simulink model "METI_Thermal_ver01_Jmaab_2018b_Intg_Mref"  (R2018b)
settings: Solver=ode8  StartTime=0  StopTime=end_time  FixedStep=sampling_time  RelTol=1e-3
PreLoadFcn:
  | %init_setting;
values from neighbouring files (symbols this model uses):
  degC2K = 273.15    [METI_TRAMI_Thermal_ver01_Jmaab_PreLoad.m]    (also in init_setting_METI.m)
  K2degC = -273.15    [METI_TRAMI_Thermal_ver01_Jmaab_PreLoad.m]    (also in init_setting_METI.m)
  sampling_time = 0.0025    [METI_TRAMI_Thermal_ver01_Jmaab_PreLoad.m]
undefined symbols (not defined in the file or in its folder): ACC_D_Gain, ACC_I_Gain, ACC_P_Gain, ALT_CNT_ALT_OFF_RPM_HYS_rpm, ALT_CNT_ALT_ON_RPM_HYS_rpm, ALT_CNT_Alter_V_BASE_V, ALT_CNT_Alter_V_Kaisei_V, ALT_CNT_flag_disable_kaisei, ALT_CNT_V_Battely_Kudo_V, ALT_PNT_ALT_GDCurrent_A, ALT_PNT_ALT_GDVolt_V, ALT_PNT_Alter_limit_Current_V_table, ALT_PNT_Alter_limit_Current_V_table_x_rpm, ALT_PNT_Alter_trq_Nm_map, ALT_PNT_Alter_trq_Nm_map_x_rpm, ALT_PNT_Alter_trq_Nm_map_y_Current_A, ALT_PNT_Alter_trq_Nm_map_z_Volt_tgt_V, ALT_PNT_eta_pulley_alt, ALT_PNT_Gain_Alt_v_del, ALT_PNT_ratio_pulley_alt, ALT_PNT_Tau_Alternator_V_tgt_s, ALT_PNT_trq_alter_output_LL_Nm, BK_PNT_Pow_UL, BK_PNT_Tau_brake, Brk_LL, Brk_PGain, Brk_UL, BT_PNT_Lo_Capa_lo_batt_F, BT_PNT_Lo_ocv_SOC_lo_batt_OCV_V_table, BT_PNT_Lo_ocv_SOC_lo_batt_OCV_V_table_x_SOC, BT_PNT_Lo_R_lo_batt_ohm, BT_PNT_Lo_SOC_MAX_lo_batt, BT_PNT_Lo_SOC_MIN_lo_batt, BT_PNT_Lo_SOC_START_lo_batt, BT_PNT_Lo_V_start_ocv, DF_PNT_DF_gear, DF_PNT_Outtemp_degC, Driver_Brake_Const1, Driver_Brake_Const3, Driver_Brake_Switch_Const2, Driver_Brk_sh, drivmode_ACC, drivmode_CONST, drivmode_GensokuKaisei, drivmode_GensokuRikko, drivmode_STOP, EL_PNT_R_bodyelec_lo_ohm, ENG_CNT_acc_idlestop, ENG_CNT_Accel_LL, ENG_CNT_Accel_UL, ENG_CNT_brak_idlestop, ENG_CNT_flag_idle_stop_exe, ENG_CNT_gain_p_per_isc, ENG_CNT_IdleSpeed, ENG_CNT_IdleSpeed_Const, ENG_CNT_IdleStop_flag_const, ENG_CNT_omg_eng_fuelcut_rpm, ENG_CNT_per_isc_max, ENG_CNT_per_isc_min, ENG_CNT_per_throttle_fuelcut ... (+82)
libraries: METI_Lib_vehicle_model x18, simulink x3, AZAPA_Lib_vehicle_model x1
(part 1 of 3)
settings Model: Creator=nishimura  LastModifiedBy=E00026
settings DataIOCC: LimitDataPoints=on  SaveFormat=Array  InspectSignalLogs=on
settings OptimizationCC: BlockReduction=off  BooleanDataType=off  LifeSpan=inf
settings DebuggingCC: SaveWithParameterizedLinksMsg=none  UnderspecifiedInitializationDetection=Classic  MergeDetectMultiDrivingBlocksExec=none  SignalResolutionControl=TryResolveAllWithWarning  StrictBusMsg=ErrorOnBusTreatedAsVector  SFUnexpectedBacktrackingDiag=warning  SFNoUnconditionalDefaultTransitionDiag=warning  SFExecutionAtInitializationDiag=none
settings HardwareCC: ProdBitPerPointer=32  ProdBitPerSizeT=32  ProdBitPerPtrDiffT=32  ProdLargestAtomicFloat=None  ProdIntDivRoundTo=Undefined  ProdEndianess=Unspecified  ProdWordSize=32  ProdHWDeviceType=32-bit Generic  TargetUnknown=on
settings ModelReferenceCC: PropagateSignalLabelsOutOfModel=off
settings SFSimCC: SimUseLocalCustomCode=off
settings RTWCC: RTWUseLocalCustomCode=off
settings CodeAppCC: StateflowObjectComments=on
settings GRTTargetCC: TargetLangStandard=C89/C90 (ANSI)  GeneratePreprocessorConditionals=Disable all
settings ConfigComp: CovMetricSettings=dw  CovHtmlReporting=on  CovSaveCumulativeToWorkspaceVar=on  CovSaveSingleToWorkspaceVar=on  CovExternalEMLEnable=off  CovSFcnEnable=off

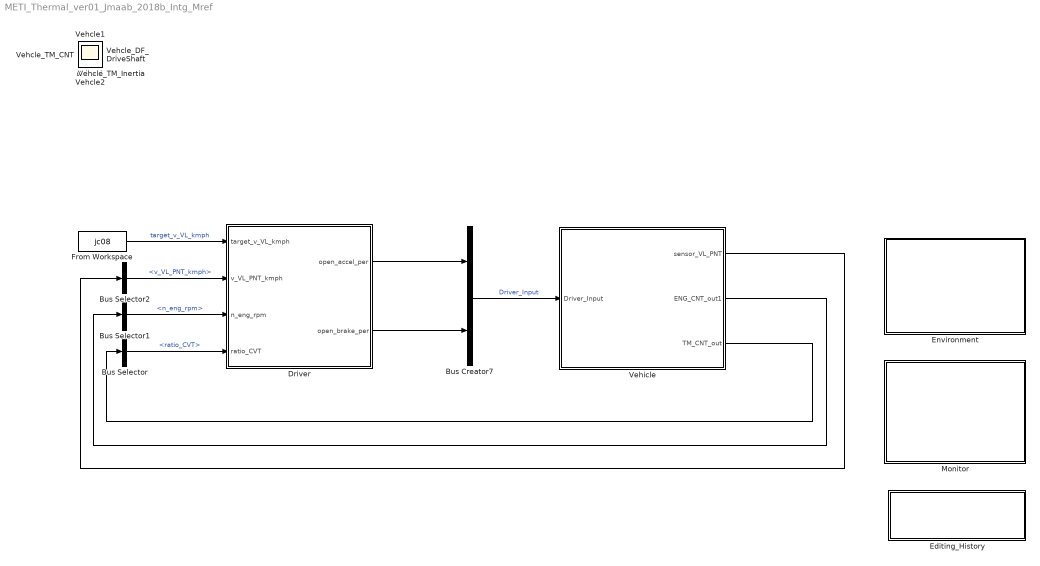
== system METI_Thermal_ver01_Jmaab_2018b_Intg_Mref ==
  Bus Creator7 : BusCreator  Inputs=2
  Bus Selector : BusSelector  OutputSignals=ratio_CVT
  Bus Selector1 : BusSelector  OutputSignals=n_eng_rpm
  Bus Selector2 : BusSelector  OutputSignals=v_VL_PNT_kmph
  Driver : Subsystem
      mask Display: image(imread('picture\ドライバ.png'))
  Editing_History : Subsystem
  Environment : Subsystem
      mask Display: image(imread('picture\外部環境.png'))
  From Workspace : FromWorkspace  VariableName=jc08  SampleTime=0  OutputAfterFinalValue=Holding final value
  Monitor : Subsystem
  Vehicle : Subsystem
      mask Display: image(imread('picture\電気負荷.png'))
  Driver1 : Scope
  Vehcle1 : Scope
  Vehcle2 : Scope
  Vehcle_DF_DriveShaft : Scope
  Vehcle_TM_CNT : Scope
  Vehcle_TM_Inertia : Scope
  wires:
  From Workspace/1 -> Driver/1(target_v_VL_kmph)  "target_v_VL_kmph"
  Bus Creator7/1 -> Vehicle/1(Driver_Input)  "Driver_Input"
  Vehicle/1(sensor_VL_PNT) -> Bus Selector2/1
  Vehicle/3(TM_CNT_out) -> Bus Selector/1
  Vehicle/2(ENG_CNT_out1) -> Bus Selector1/1
  Driver/1(open_accel_per) -> Bus Creator7/1
  Driver/2(open_brake_per) -> Bus Creator7/2
  Bus Selector/1 -> Driver/4(ratio_CVT)  "<ratio_CVT>"
  Bus Selector1/1 -> Driver/3(n_eng_rpm)  "<n_eng_rpm>"
  Bus Selector2/1 -> Driver/2(v_VL_PNT_kmph)  "<v_VL_PNT_kmph>"

== system METI_Thermal_ver01_Jmaab_2018b_Intg_Mref/Driver ==
  note: ドライバモデルのへたくそ対応
  note: 全体としてパワーを算出しておいて、
      | さらにパワーと速度のF/Bを切り替えれるようにしておく
  target_v_VL_kmph : Inport
  v_VL_PNT_kmph : Inport  Port=2
  n_eng_rpm : Inport  Port=3
  ratio_CVT : Inport  Port=4
  Caliculate_Driving_State : Subsystem
  Caliculate_Opeining_Accel : Subsystem
  Caliculate_Opening_Brake : Subsystem
  Memory2 : Memory  InheritSampleTime=on
  Memory3 : Memory
  Memory4 : Memory
  open_accel_per : Outport
  open_brake_per : Outport  Port=2
  tag scope: tScope_accel=global, tScope_brake=global
  wires:
  target_v_VL_kmph/1 -> Caliculate_Opening_Brake/2(target_v_VL_kmph), Caliculate_Driving_State/2(target_v_VL_kmph), Caliculate_Opeining_Accel/2(target_v_VL_kmph)
  Memory3/1 -> Caliculate_Opeining_Accel/3(pre_n_eng_rpm)  "pre_n_eng_rpm"
  ratio_CVT/1 -> Memory4/1
  Memory4/1 -> Caliculate_Opeining_Accel/4(pre_ratio_CVT)  "pre_ratio_CVT"
  n_eng_rpm/1 -> Memory3/1
  Memory2/1 -> Caliculate_Opening_Brake/1(v_VL_PNT_kmph), Caliculate_Opeining_Accel/1(v_VL_PNT_kmph)
  Caliculate_Opeining_Accel/1(open_accel_per) -> Caliculate_Opening_Brake/3(open_accel_per), open_accel_per/1, [tScope_accel]
  Caliculate_Opening_Brake/1(open_brake_per) -> Caliculate_Driving_State/1(open_brake_per), open_brake_per/1, [tScope_brake]
  v_VL_PNT_kmph/1 -> Memory2/1

== system METI_Thermal_ver01_Jmaab_2018b_Intg_Mref/Editing_History ==
  note: 編集履歴
      |
      | 2019/3/29　初版
      |
      | 2019/7/3　ver.2
      | ・ENG_CNT内部と出力の結線名を修正
      | ・DFとPTTH間の熱のI/Fを追加修正
      | ・PTTH_PNT/RDTH_PNTの絵が同梱されていなかったため追加

== system METI_Thermal_ver01_Jmaab_2018b_Intg_Mref/Environment ==
  note: 登坂。風、温度、湿度・・・
  Clock : Clock
  To Workspace : ToWorkspace  VariableName=simtime  SampleTime=-1
      settings: Decimation=num_tws_mabiki
  wires:
  Clock/1 -> To Workspace/1

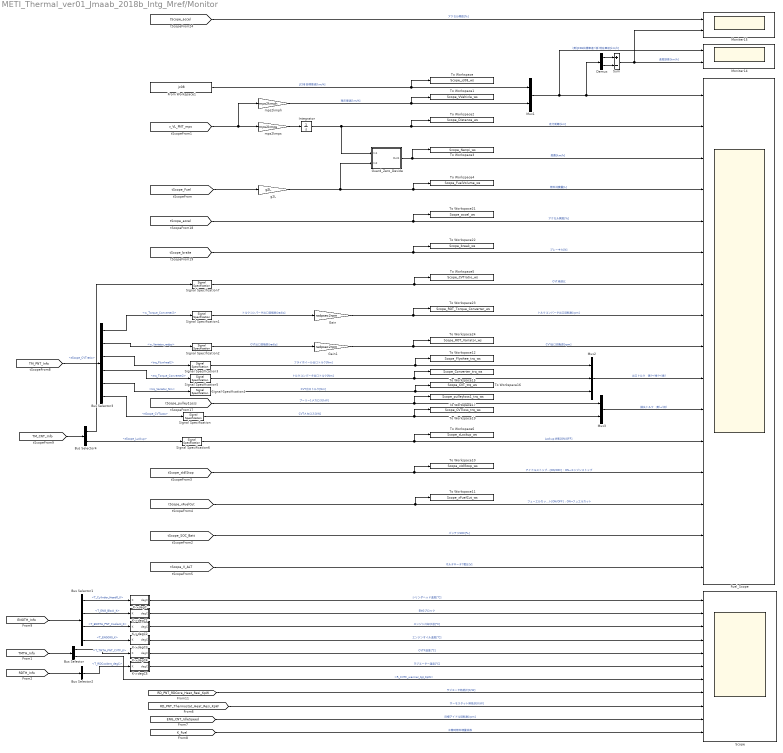
== system METI_Thermal_ver01_Jmaab_2018b_Intg_Mref/Monitor ==
  Bus Selector : BusSelector  OutputSignals=T_TMTH_PNT_CVTF_K,R_CVTF_warmer_tgt_KpW
  Bus Selector1 : BusSelector  OutputSignals=T_Cylinder_Head0_K,T_ENG_Block_K,T_ENGTH_PNT_Coolant_K,T_ENGOil0_K
  Bus Selector2 : BusSelector  OutputSignals=T_RDCoolant_degC
  Bus Selector3 : BusSelector  OutputSignals=w_Torque_Converter2,w_Variator_radps,trq_Flywheel2,trq_Torque_Converter2,trq_Variator_Nm,tScope_CVTLoss
  Bus Selector4 : BusSelector  OutputSignals=tScope_CVTratio,tScope_Luckup
  Demux : Demux  Outputs=2
  From Workspace1 : FromWorkspace  VariableName=jc08  SampleTime=0  OutputAfterFinalValue=Holding final value
  Fuel_Scope : Scope  NumInputPorts=16
  Gain : Gain  Gain=radpsec2rpm
  Gain1 : Gain  Gain=radpsec2rpm
  Guard_Zero_Devide : Subsystem
  Integrator : Integrator
  K->degC : Subsystem
  K->degC1 : Subsystem
  K->degC2 : Subsystem
  K->degC3 : Subsystem
  K->degC4 : Subsystem
  K->degC5 : Subsystem
  Moniter14 : Scope  NumInputPorts=2
  Moniter15 : Scope  NumInputPorts=2
  Mux1 : Mux  Inputs=2
  Mux2 : Mux  Inputs=3
  Mux3 : Mux  Inputs=2
  Scope : Scope  NumInputPorts=11
  Signal Specification{,1..7} (8 alike) : SignalSpecification
  Sum : Sum  Inputs=+-
  To Workspace : ToWorkspace  VariableName=Scope_jc08_ws  SaveFormat=Structure With Time  SampleTime=-1
      settings: Decimation=num_tws_mabiki
  To Workspace1 : ToWorkspace  VariableName=Scope_VVehicle_ws  SaveFormat=Structure With Time  SampleTime=-1
      settings: Decimation=num_tws_mabiki
  To Workspace10 : ToWorkspace  VariableName=Scope_xIdlStop_ws  SaveFormat=Structure With Time  SampleTime=-1
      settings: Decimation=num_tws_mabiki
  To Workspace11 : ToWorkspace  VariableName=Scope_xFuelCut_ws  SaveFormat=Structure With Time  SampleTime=-1
      settings: Decimation=num_tws_mabiki
  To Workspace12 : ToWorkspace  VariableName=Scope_Flywhee_trq_ws  SaveFormat=Structure With Time  SampleTime=-1
      settings: Decimation=num_tws_mabiki
  To Workspace15 : ToWorkspace  VariableName=Scope_Converter_trq_ws  SaveFormat=Structure With Time  SampleTime=-1
      settings: Decimation=num_tws_mabiki
  To Workspace16 : ToWorkspace  VariableName=Scope_CVT_trq_ws  SaveFormat=Structure With Time  SampleTime=-1
      settings: Decimation=num_tws_mabiki
  To Workspace17 : ToWorkspace  VariableName=Scope_pulleyloss1_trq_ws  SaveFormat=Structure With Time  SampleTime=-1
      settings: Decimation=num_tws_mabiki
  To Workspace19 : ToWorkspace  VariableName=Scope_CVTloss_trq_ws  SaveFormat=Structure With Time  SampleTime=-1
      settings: Decimation=num_tws_mabiki
  To Workspace2 : ToWorkspace  VariableName=Scope_Distance_ws  SaveFormat=Structure With Time  SampleTime=-1
      settings: Decimation=num_tws_mabiki
  To Workspace21 : ToWorkspace  VariableName=Scope_accel_ws  SaveFormat=Structure With Time  SampleTime=-1
      settings: Decimation=num_tws_mabiki
  To Workspace22 : ToWorkspace  VariableName=Scope_break_ws  SaveFormat=Structure With Time  SampleTime=-1
      settings: Decimation=num_tws_mabiki
  To Workspace23 : ToWorkspace  VariableName=Scope_ROT_Torque_Converter_ws  SaveFormat=Structure With Time  SampleTime=-1
      settings: Decimation=num_tws_mabiki
  To Workspace24 : ToWorkspace  VariableName=Scope_ROT_Variator_ws  SaveFormat=Structure With Time  SampleTime=-1
      settings: Decimation=num_tws_mabiki
  To Workspace3 : ToWorkspace  VariableName=Scope_Nenpi_ws  SaveFormat=Structure With Time  SampleTime=-1
      settings: Decimation=num_tws_mabiki
  To Workspace4 : ToWorkspace  VariableName=Scope_FuelVolume_ws  SaveFormat=Structure With Time  SampleTime=-1
      settings: Decimation=num_tws_mabiki
  To Workspace5 : ToWorkspace  VariableName=Scope_CVTratio_ws  SaveFormat=Structure With Time  SampleTime=-1
      settings: Decimation=num_tws_mabiki
  To Workspace6 : ToWorkspace  VariableName=Scope_xLockup_ws  SaveFormat=Structure With Time  SampleTime=-1
      settings: Decimation=num_tws_mabiki
  g2L : Gain  Gain=g2L
  mps2kmph : Gain  Gain=mps2kmph
  mps2kmps : Gain  Gain=mps2kmps
  wires:
  [tScope_xIdlStop] -> To Workspace10/1, Fuel_Scope/13  "アイドルストップ[ON/OFF] : ON→エンジンストップ"
  [tScope_xFuelCut] -> To Workspace11/1, Fuel_Scope/14  "フューエルカット[ON/OFF] : ON→フュエルカット"
  [v_VL_PNT_mps] -> mps2kmph/1, mps2kmps/1
  mps2kmps/1 -> Integrator/1
  [tScope_Fuel] -> g2L/1
  Integrator/1 -> Guard_Zero_Devide/1(In1), To Workspace2/1, Fuel_Scope/2  "走行距離[km]"
  g2L/1 -> To Workspace4/1, Fuel_Scope/4, Guard_Zero_Devide/2(In2)  "燃料消費量[L]"
  Signal Specification6/1 -> To Workspace6/1, Fuel_Scope/12  "Lockup状態[ON/OFF]"
  Signal Specification7/1 -> To Workspace5/1, Fuel_Scope/7  "CVT減速比"
  From Workspace1/1 -> To Workspace/1, Mux1/1  "JC08目標車速[km/h]"
  mps2kmph/1 -> To Workspace1/1, Mux1/2  "現在車速[km/h]"
  Mux1/1 -> Moniter14/1, Demux/1, Fuel_Scope/1  "(黄)JC08目標車速/(桃)現在車速[km/h]"
  Signal Specification/1 -> To Workspace19/1, Mux3/2  "CVTメカロス[kW]"
  Signal Specification3/1 -> To Workspace12/1, Mux2/1  "フライホイール出口トルク[Nm]"
  Signal Specification5/1 -> To Workspace15/1, Mux2/2  "トルクコンバータ出口トルク[Nm]"
  Signal Specification4/1 -> To Workspace16/1, Mux2/3  "CVT出口トルク[Nm]"
  [tScope_pulley1Loss] -> To Workspace17/1, Mux3/1  "プーリー1メカロス[kW]"
  Mux2/1 -> Fuel_Scope/10  "出口トルク  (黄)→(桃)→(青)"
  Mux3/1 -> Fuel_Scope/11  "損失トルク  (黄)→(桃)"
  [tScope_accel] -> To Workspace21/1, Fuel_Scope/5  "アクセル開度[%]"
  [tScope_brake] -> To Workspace22/1, Fuel_Scope/6  "ブレーキ力[N]"
  Gain/1 -> Fuel_Scope/8, To Workspace23/1  "トルクコンバータ出口回転数[rpm]"
  Signal Specification2/1 -> Gain1/1  "CVT出口回転数[rad/s]"
  Demux/1 -> Sum/1
  Demux/2 -> Sum/2
  Sum/1 -> Moniter14/2, Moniter15/2  "速度誤差[km/h]"
  [tScope_accel] -> Moniter15/1  "アクセル開度[%]"
  [tScope_V_ALT] -> Fuel_Scope/16  "オルタネータ7電圧[V]"
  [tScope_SOC_Batt] -> Fuel_Scope/15  "バッテリSOC[%]"
  Guard_Zero_Devide/1(Out1) -> To Workspace3/1, Fuel_Scope/3  "燃費[km/h]"
  K->degC4/1(degC) -> Scope/5  "CVTF温度[℃]"
  K->degC5/1(degC) -> Scope/6  "ラジエーター温度[℃]"
  K->degC2/1(degC) -> Scope/3  "エンジン冷却水温[℃]"
  K->degC3/1(degC) -> Scope/4  "エンジンオイル温度[℃]"
  K->degC/1(degC) -> Scope/1  "シリンダヘッド温度[℃]"
  K->degC1/1(degC) -> Scope/2  "ENGブロック"
  Signal Specification1/1 -> Gain/1  "トルクコンバータ出口回転数[rad/s]"
  Gain1/1 -> To Workspace24/1, Fuel_Scope/9  "CVT出口回転数[rpm]"
  [RD_PNT_RDCore_Heat_Resi_KpW] -> Scope/8  "ラジエータ熱抵抗[K/W]"
  [RD_PNT_Thermostat_Heat_Resi_KpW] -> Scope/9  "サーモスタット熱抵抗[K/W]"
  [ENG_CNT_IdleSpeed] -> Scope/10  "目標アイドル回転数[rpm]"
  [K_Fuel] -> Scope/11  "冷機時燃料増量係数"
  [ENGTH_Info] -> Bus Selector1/1
  Bus Selector1/1 -> K->degC/1(K)  "<T_Cylinder_Head0_K>"
  Bus Selector1/2 -> K->degC1/1(K)  "<T_ENG_Block_K>"
  Bus Selector1/3 -> K->degC2/1(K)  "<T_ENGTH_PNT_Coolant_K>"
  Bus Selector1/4 -> K->degC3/1(K)  "<T_ENGOil0_K>"
  [TMTH_Info] -> Bus Selector/1
  Bus Selector/1 -> K->degC4/1(K)  "<T_TMTH_PNT_CVTF_K>"
  [RDTH_Info] -> Bus Selector2/1
  Bus Selector2/1 -> K->degC5/1(K)  "<T_RDCoolant_degC>"
  Bus Selector/2 -> Scope/7  "<R_CVTF_warmer_tgt_KpW>"
  [TM_PNT_Info] -> Bus Selector3/1
  Bus Selector3/6 -> Signal Specification/1  "<tScope_CVTLoss>"
  Bus Selector3/1 -> Signal Specification1/1  "<w_Torque_Converter2>"
  Bus Selector3/2 -> Signal Specification2/1  "<w_Variator_radps>"
  Bus Selector3/3 -> Signal Specification3/1  "<trq_Flywheel2>"
  Bus Selector3/5 -> Signal Specification4/1  "<trq_Variator_Nm>"
  Bus Selector3/4 -> Signal Specification5/1  "<trq_Torque_Converter2>"
  [TM_CNT_Info] -> Bus Selector4/1
  Bus Selector4/2 -> Signal Specification6/1  "<tScope_Luckup>"
  Bus Selector4/1 -> Signal Specification7/1  "<tScope_CVTratio>"

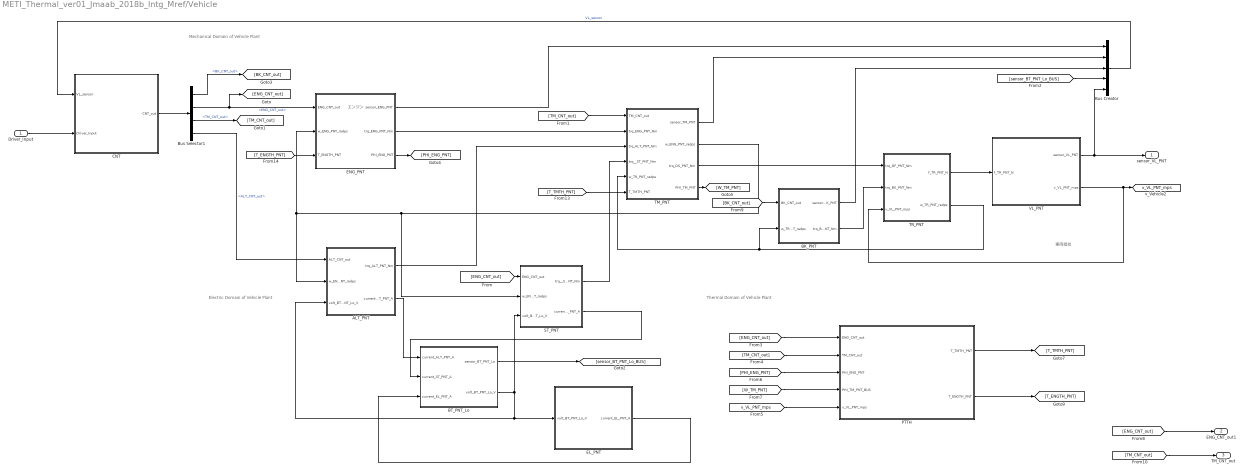
== system METI_Thermal_ver01_Jmaab_2018b_Intg_Mref/Vehicle ==
  note: Thermal Domain of Vehicle Plant
  note: エンジン
  note: 車両抵抗
  note: Mechanical Domain of Vehicle Plant
  note: Electric Domain
      |  of Vehicle Plant
  Driver_Input : Inport
  ALT_PNT : Subsystem
      mask Display: image(imread('picture\image\オルタネータ02.jpg'))
  BK_PNT : Subsystem
      mask Display: image(imread('picture\ブレーキ02.png'))
  BT_PNT_Lo : Subsystem
      mask Display: image(imread('picture\バッテリー.png'))
  Bus Creator : BusCreator  Inputs=5
  Bus Selector1 : BusSelector  OutputSignals=BK_CNT_out,ENG_CNT_out,TM_CNT_out,ALT_CNT_out
  CNT : Subsystem
      mask Display: image(imread('picture\ECU.png'))
  EL_PNT : Subsystem
      mask Display: image(imread('picture\電気負荷.png'))
  ENG_PNT : Subsystem
      mask Display: image(imread('picture\image\エンジン03.jpg'))
  PTTH : Subsystem
  ST_PNT : Subsystem
      mask Display: image(imread('picture\image\スターター02.jpg'))
  TM_PNT : Subsystem
      mask Display: image(imread('picture\image\トランスミッション02.jpg'))
  TR_PNT : Subsystem
      mask Display: image(imread('picture\タイヤ01.png'))
  VL_PNT : Subsystem
      mask Display: image(imread('picture\車両抵抗.png'))
  sensor_VL_PNT : Outport
  ENG_CNT_out1 : Outport  Port=2
  TM_CNT_out : Outport  Port=3
  tag scope: v_VL_PNT_mps=global
  wires:
  ALT_PNT/1(trq_ALT_PNT_Nm) -> TM_PNT/3(trq_ALT_PNT_Nm)
  EL_PNT/1(current_EL_PNT_A) -> BT_PNT_Lo/3(current_EL_PNT_A)
  ALT_PNT/2(current_ALT_PNT_A) -> BT_PNT_Lo/1(current_ALT_PNT_A)
  ST_PNT/2(current_ST_PNT_A) -> BT_PNT_Lo/2(current_ST_PNT_A)
  BT_PNT_Lo/2(volt_BT_PNT_Lo_V) -> ST_PNT/3(volt_BT_PNT_Lo_V), ALT_PNT/3(volt_BT_PNT_Lo_V), EL_PNT/1(volt_BT_PNT_Lo_V)
  ENG_PNT/2(trq_ENG_PNT_Nm) -> TM_PNT/2(trq_ENG_PNT_Nm)
  ST_PNT/1(trq__ST_PNT_Nm) -> TM_PNT/4(trq__ST_PNT_Nm)
  VL_PNT/1(sensor_VL_PNT) -> Bus Creator/5, sensor_VL_PNT/1
  BK_PNT/2(trq_BK_PNT_Nm) -> TR_PNT/2(trq_BK_PNT_Nm)
  TR_PNT/1(f_TR_PNT_N) -> VL_PNT/1(f_TR_PNT_N)
  TR_PNT/2(w_TR_PNT_radps) -> BK_PNT/2(w_TR_PNT_radps), TM_PNT/5(w_TR_PNT_radps)
  VL_PNT/2(v_VL_PNT_mps) -> TR_PNT/3(v_VL_PNT_mps), [v_VL_PNT_mps]
  [TM_CNT_out] -> TM_CNT_out/1
  Bus Selector1/2 -> [ENG_CNT_out], ENG_PNT/1(ENG_CNT_out)  "<ENG_CNT_out>"
  Bus Selector1/4 -> ALT_PNT/1(ALT_CNT_out)  "<ALT_CNT_out>"
  CNT/1(CNT_out) -> Bus Selector1/1
  [ENG_CNT_out] -> ST_PNT/1(ENG_CNT_out)
  Bus Selector1/3 -> [TM_CNT_out]  "<TM_CNT_out>"
  [TM_CNT_out] -> TM_PNT/1(TM_CNT_out)
  BT_PNT_Lo/1(sensor_BT_PNT_Lo) -> [sensor_BT_PNT_Lo_BUS]
  Driver_Input/1 -> CNT/2(Driver_Input)
  [ENG_CNT_out] -> ENG_CNT_out1/1
  TM_PNT/3(trq_DS_PNT_Nm) -> TR_PNT/1(trq_DF_PNT_Nm)
  [T_TMTH_PNT] -> TM_PNT/6(T_TMTH_PNT)
  [v_VL_PNT_mps] -> PTTH/5(v_VL_PNT_mps)
  [ENG_CNT_out] -> PTTH/1(ENG_CNT_out)
  [TM_CNT_out] -> PTTH/2(TM_CNT_out)
  ENG_PNT/3(PHI_ENG_PNT) -> [PHI_ENG_PNT]
  [PHI_ENG_PNT] -> PTTH/3(PHI_ENG_PNT)
  [W_TM_PNT] -> PTTH/4(PHI_TM_PNT_BUS)
  TM_PNT/4(PHI_TM_PNT) -> [W_TM_PNT]
  PTTH/1(T_TMTH_PNT) -> [T_TMTH_PNT]
  PTTH/2(T_ENGTH_PNT) -> [T_ENGTH_PNT]
  [T_ENGTH_PNT] -> ENG_PNT/3(T_ENGTH_PNT)
  [sensor_BT_PNT_Lo_BUS] -> Bus Creator/4
  ENG_PNT/1(sensor_ENG_PNT) -> Bus Creator/1
  TM_PNT/1(sensor_TM_PNT) -> Bus Creator/2
  Bus Selector1/1 -> [BK_CNT_out]  "<BK_CNT_out>"
  [BK_CNT_out] -> BK_PNT/1(BK_CNT_out)
  Bus Creator/1 -> CNT/1(VL_sensor)  "VL_sensor"
  TM_PNT/2(w_ENG_PNT_radps) -> ENG_PNT/2(w_ENG_PNT_radps), ALT_PNT/2(w_ENG_PNT_radps), ST_PNT/2(w_ENG_PNT_radps)
  BK_PNT/1(sensor_BK_PNT) -> Bus Creator/3

== system METI_Thermal_ver01_Jmaab_2018b_Intg_Mref/Driver/Caliculate_Driving_State ==
  open_brake_per : Inport
  target_v_VL_kmph : Inport  Port=2
  Constant : Constant  Value=Thresh_Stop_vCar
  Constant4 : Constant  Value=0.1*sampling_time
  Constant6 : Constant  Value=-0.1*sampling_time
  Memory : Memory
  Relational Operator : RelationalOperator  Operator=>  OutDataTypeStr=boolean  RndMeth=Nearest
  Relational Operator1 : RelationalOperator  Operator=<  OutDataTypeStr=boolean  RndMeth=Nearest
  Relational Operator2 : RelationalOperator  Operator=<  OutDataTypeStr=boolean  RndMeth=Nearest
  Sum : Sum  Inputs=|+-
  Switch{,1..3} (4 alike) : Switch  Criteria=u2 > Threshold  Threshold=0.5
  Terminator : Terminator
  停止 : Constant  Value=drivmode_STOP
  加速 : Constant  Value=drivmode_ACC
  定常1 : Constant  Value=drivmode_CONST
  減速力行 : Constant  Value=drivmode_GensokuRikko
  減速回生 : Constant  Value=drivmode_GensokuKaisei
  wires:
  Switch/1 -> Terminator/1  "state_driving"
  target_v_VL_kmph/1 -> Relational Operator/1, Memory/1, Sum/1
  Relational Operator1/1 -> Switch1/2
  Constant4/1 -> Relational Operator1/2
  Relational Operator/1 -> Switch/2
  Constant/1 -> Relational Operator/2
  停止/1 -> Switch/3
  Sum/1 -> Relational Operator1/1, Relational Operator2/1
  減速回生/1 -> Switch2/1
  Switch3/1 -> Switch1/1
  Constant6/1 -> Relational Operator2/2
  Memory/1 -> Sum/2
  open_brake_per/1 -> Switch2/2
  減速力行/1 -> Switch2/3
  Relational Operator2/1 -> Switch3/2
  Switch2/1 -> Switch3/1
  定常1/1 -> Switch3/3
  加速/1 -> Switch1/3
  Switch1/1 -> Switch/1

== system METI_Thermal_ver01_Jmaab_2018b_Intg_Mref/Driver/Caliculate_Opeining_Accel ==
  v_VL_PNT_kmph : Inport
  target_v_VL_kmph : Inport  Port=2
  pre_n_eng_rpm : Inport  Port=3
  pre_ratio_CVT : Inport  Port=4
  FB : Subsystem  mask{P_Gain=ACC_P_Gain, D_Gain=ACC_D_Gain, I_Gain=ACC_I_Gain}
      mask prompts: P_Gain "Pゲイン値"; D_Gain "Dゲイン値"; I_Gain "Iゲイン値"
  FF : Subsystem
  Guard_0_100 : Saturate  UpperLimit=ENG_CNT_Throttle_UL  LowerLimit=ENG_CNT_Throttle_LL
  Sum1 : Sum  Inputs=|-+
  Sum3 : Sum  Inputs=++|
  open_accel_per : Outport
  wires:
  Sum1/1 -> FB/1(delta_v_VL_kmph)
  v_VL_PNT_kmph/1 -> FF/1(v_VL_PNT_kmph), Sum1/1
  target_v_VL_kmph/1 -> FF/2(target_v_VL_kmph), Sum1/2
  Sum3/1 -> Guard_0_100/1
  pre_n_eng_rpm/1 -> FF/3(pre_n_eng_rpm)
  pre_ratio_CVT/1 -> FF/4(pre_ratio_CVT)
  FB/1(FB_open_accel_per) -> Sum3/1
  FF/1(FF_open_accel_per) -> Sum3/2
  Guard_0_100/1 -> open_accel_per/1  "open_accel_per"

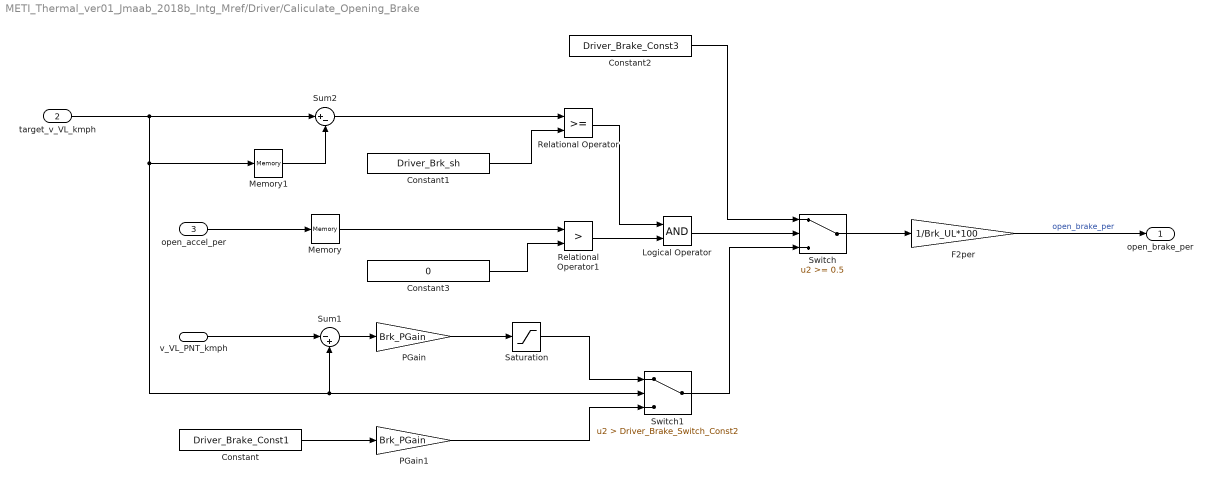
== system METI_Thermal_ver01_Jmaab_2018b_Intg_Mref/Driver/Caliculate_Opening_Brake ==
  v_VL_PNT_kmph : Inport
  target_v_VL_kmph : Inport  Port=2
  open_accel_per : Inport  Port=3
  Constant : Constant  Value=Driver_Brake_Const1
  Constant1 : Constant  Value=Driver_Brk_sh
  Constant2 : Constant  Value=Driver_Brake_Const3
  Constant3 : Constant  Value=0
  F2per : Gain  Gain=1/Brk_UL*100
  Logical Operator : Logic  AllPortsSameDT=off  OutDataTypeStr=boolean
  Memory : Memory
  Memory1 : Memory
  PGain : Gain  Gain=Brk_PGain
  PGain1 : Gain  Gain=Brk_PGain
  Relational Operator : RelationalOperator  OutDataTypeStr=boolean  RndMeth=Nearest
  Relational Operator1 : RelationalOperator  Operator=>  OutDataTypeStr=boolean  RndMeth=Nearest
  Saturation : Saturate  UpperLimit=Brk_UL  LowerLimit=Brk_LL
  Sum1 : Sum  Inputs=|-+
  Sum2 : Sum  Inputs=|+-
  Switch : Switch  Threshold=0.5
  Switch1 : Switch  Criteria=u2 > Threshold  Threshold=Driver_Brake_Switch_Const2
  open_brake_per : Outport
  wires:
  target_v_VL_kmph/1 -> Switch1/2, Sum1/2, Memory1/1, Sum2/1
  Sum1/1 -> PGain/1
  PGain/1 -> Saturation/1
  Constant/1 -> PGain1/1
  PGain1/1 -> Switch1/3
  open_accel_per/1 -> Memory/1
  Memory/1 -> Relational Operator1/1
  Memory1/1 -> Sum2/2
  Switch/1 -> F2per/1
  Sum2/1 -> Relational Operator/1
  Saturation/1 -> Switch1/1
  Switch1/1 -> Switch/3
  Constant2/1 -> Switch/1
  v_VL_PNT_kmph/1 -> Sum1/1
  Constant1/1 -> Relational Operator/2
  Constant3/1 -> Relational Operator1/2
  Relational Operator1/1 -> Logical Operator/2
  Relational Operator/1 -> Logical Operator/1
  Logical Operator/1 -> Switch/2
  F2per/1 -> open_brake_per/1  "open_brake_per"

== system METI_Thermal_ver01_Jmaab_2018b_Intg_Mref/Monitor/Guard_Zero_Devide ==
  note: 0割防止暫定処置
  In1 : Inport
  In2 : Inport  Port=2
  Constant1 : Constant  Value=fuel_0guard
  Constant2 : Constant  Value=fuelcomsnp_0
  Divide : Product  Inputs=*/
  MinMax : MinMax  Function=max  Inputs=2
  Relational Operator : RelationalOperator  OutDataTypeStr=boolean  RndMeth=Nearest
  Switch1 : Switch  Criteria=u2 > Threshold  Threshold=0.5
  Out1 : Outport
  wires:
  In2/1 -> MinMax/1, Relational Operator/1
  In1/1 -> Divide/1
  Switch1/1 -> Out1/1  "燃費[km/l]"
  Divide/1 -> Switch1/1  "燃費[km/l]"
  Constant2/1 -> Switch1/3
  Relational Operator/1 -> Switch1/2
  MinMax/1 -> Divide/2
  Constant1/1 -> MinMax/2, Relational Operator/2

== system METI_Thermal_ver01_Jmaab_2018b_Intg_Mref/Monitor/K->degC ==
  K : Inport
  Constant2 : Constant  Value=K2degC
  Sum : Sum  Inputs=++|
  degC : Outport
  wires:
  Sum/1 -> degC/1
  Constant2/1 -> Sum/1
  K/1 -> Sum/2

== system METI_Thermal_ver01_Jmaab_2018b_Intg_Mref/Monitor/K->degC1 ==
  K : Inport
  Constant2 : Constant  Value=K2degC
  Sum : Sum  Inputs=++|
  degC : Outport
  wires:
  K/1 -> Sum/2
  Constant2/1 -> Sum/1
  Sum/1 -> degC/1

== system METI_Thermal_ver01_Jmaab_2018b_Intg_Mref/Monitor/K->degC2 ==
  K : Inport
  Constant2 : Constant  Value=K2degC
  Sum : Sum  Inputs=++|
  degC : Outport
  wires:
  Sum/1 -> degC/1
  Constant2/1 -> Sum/1
  K/1 -> Sum/2

== system METI_Thermal_ver01_Jmaab_2018b_Intg_Mref/Monitor/K->degC3 ==
  K : Inport
  Constant2 : Constant  Value=K2degC
  Sum : Sum  Inputs=++|
  degC : Outport
  wires:
  K/1 -> Sum/2
  Constant2/1 -> Sum/1
  Sum/1 -> degC/1

== system METI_Thermal_ver01_Jmaab_2018b_Intg_Mref/Monitor/K->degC4 ==
  K : Inport
  Constant2 : Constant  Value=K2degC
  Sum : Sum  Inputs=++|
  degC : Outport
  wires:
  Sum/1 -> degC/1
  Constant2/1 -> Sum/1
  K/1 -> Sum/2

== system METI_Thermal_ver01_Jmaab_2018b_Intg_Mref/Monitor/K->degC5 ==
  K : Inport
  Constant2 : Constant  Value=K2degC
  Sum : Sum  Inputs=++|
  degC : Outport
  wires:
  K/1 -> Sum/2
  Constant2/1 -> Sum/1
  Sum/1 -> degC/1

== system METI_Thermal_ver01_Jmaab_2018b_Intg_Mref/Vehicle/ALT_PNT ==
  note: 発電する為のトルクが負
  note: スルー量が出力の場合、発電する方向が正
  ALT_CNT_out : Inport
  w_ENG_PNT_radps : Inport  Port=2
  volt_BT_PNT_Lo_V : Inport  Port=3
  Bus Selector8 : BusSelector  OutputSignals=target_volt_ALT_V
  Gain : Gain  Gain=-1
  Memory1 : Memory
  P_cal : METI_Lib_vehicle_model/P_cal  Type_energy=回転運動  Type_output_energy=出力  Power_name=Po_  t_Workspace_Name=ALT_PNT_MECK  P_VariableName=Po_ALT_PNT_MECK  Across_VariableName=w_ALT_PNT_MECK  Throgh_VariableName=tq_ALT_PNT_MECK
  P_cal1 : METI_Lib_vehicle_model/P_cal  Type_energy=電気  Type_output_energy=出力  Power_name=Po_  t_Workspace_Name=ALT_PNT_ELEC  P_VariableName=Po_ALT_PNT_ELEC  Across_VariableName=V_ALT_PNT_ELEC  Throgh_VariableName=I_ALT_PNT_ELEC
  Subsystem : Subsystem
  Terminator : Terminator
  Terminator1 : Terminator
  pulley_slave : Subsystem
  trq_ALT_PNT_Nm : Outport
  current_ALT_PNT_A : Outport  Port=2
  tag scope: tScope_V_ALT=global
  wires:
  Memory1/1 -> Subsystem/2(w_ROT_slavepulley12)
  Subsystem/1(current_ALT_PNT_A) -> P_cal1/2, current_ALT_PNT_A/1
  Gain/1 -> trq_ALT_PNT_Nm/1  "trq_ALT_PNT_Nm"
  pulley_slave/1(trq_slavepulley11) -> Gain/1
  w_ENG_PNT_radps/1 -> pulley_slave/1(w_ENG_PNT_radps)
  Subsystem/2(trq_trqsource) -> P_cal/2, pulley_slave/2(trq_slavepulley12)
  volt_BT_PNT_Lo_V/1 -> [tScope_V_ALT], P_cal1/1, Subsystem/3(volt_BT_PNT_Lo_V)
  P_cal1/1 -> Terminator1/1
  P_cal/1 -> Terminator/1
  pulley_slave/2(w_slavepulley12) -> P_cal/1, Memory1/1
  ALT_CNT_out/1 -> Bus Selector8/1
  Bus Selector8/1 -> Subsystem/1(target_volt_ALT_V)  "<target_volt_ALT_V>"

== system METI_Thermal_ver01_Jmaab_2018b_Intg_Mref/Vehicle/BK_PNT ==
  note: 制動力
  BK_CNT_out : Inport
  w_TR_PNT_radps : Inport  Port=2
  Bus Creator : BusCreator  Inputs=1
  Bus Selector : BusSelector  OutputSignals=open_brake_per
  Constant2 : Constant  Value=tire_r
  Gain : Gain  Gain=-1
  Memory : Memory
  Product6 : Product  RndMeth=Zero
  Q_cal3 : METI_Lib_vehicle_model/P_cal  Type_energy=回転運動  Type_output_energy=損失  Power_name=Pl_  t_Workspace_Name=BK_PNT_MECK_LOSS  P_VariableName=Pl_BK_PNT_MECK_LOSS  Across_VariableName=w_BK_PNT_MECK_LOSS  Throgh_VariableName=tq_BK_PNT_MECK_LOSS
  Terminator1 : Terminator
  Transfer Fcn : TransferFcn  Denominator=[BK_PNT_Tau_brake 1]
  per2F : Gain  Gain=BK_PNT_Pow_UL/100
  sensor_BK_PNT : Outport
  trq_BK_PNT_Nm : Outport  Port=2
  wires:
  Q_cal3/1 -> Terminator1/1
  Transfer Fcn/1 -> Product6/2
  Constant2/1 -> Product6/1
  Product6/1 -> Gain/1, Q_cal3/2
  w_TR_PNT_radps/1 -> Q_cal3/1
  BK_CNT_out/1 -> Bus Selector/1
  Gain/1 -> Bus Creator/1, trq_BK_PNT_Nm/1  "trq_BK_PNT_Nm"
  per2F/1 -> Transfer Fcn/1
  Bus Selector/1 -> per2F/1  "<open_brake_per>"
  Memory/1 -> sensor_BK_PNT/1  "sensor_BK_PNT"
  Bus Creator/1 -> Memory/1

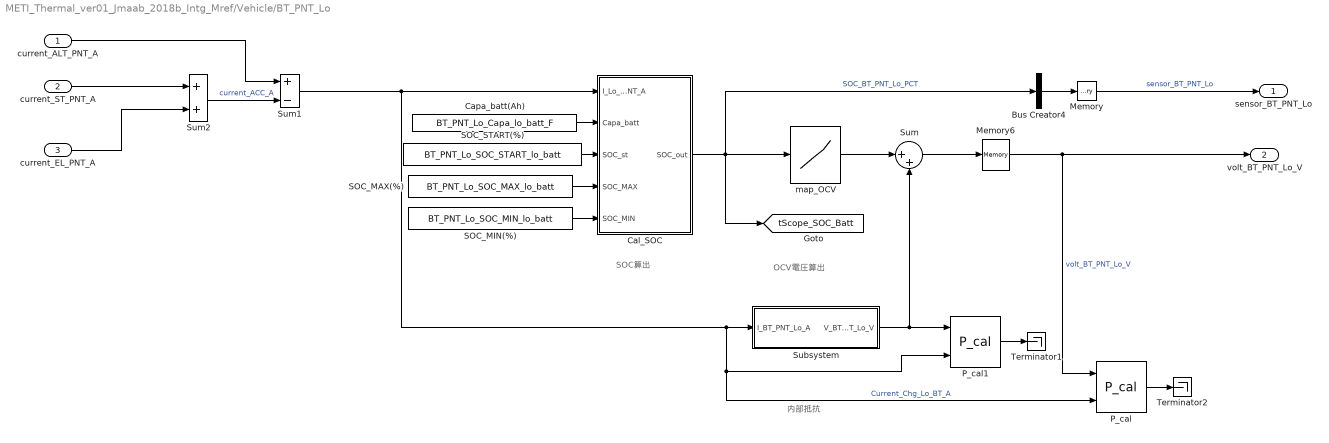
== system METI_Thermal_ver01_Jmaab_2018b_Intg_Mref/Vehicle/BT_PNT_Lo ==
  note: SOC算出
  note: 内部抵抗
  note: OCV電圧算出
  current_ALT_PNT_A : Inport
  current_ST_PNT_A : Inport  Port=2
  current_EL_PNT_A : Inport  Port=3
  Bus Creator4 : BusCreator  Inputs=1
  Cal_SOC : Subsystem
  Capa_batt(Ah) : Constant  Value=BT_PNT_Lo_Capa_lo_batt_F
  Memory : Memory
  Memory6 : Memory  InitialCondition=BT_PNT_Lo_V_start_ocv  InheritSampleTime=on
  P_cal : METI_Lib_vehicle_model/P_cal  Type_energy=電気  Type_output_energy=出力  Power_name=Po_  t_Workspace_Name=BT_PNT_Lo_ELEC  P_VariableName=Po_BT_PNT_Lo_ELEC  Across_VariableName=V_BT_PNT_Lo_ELEC  Throgh_VariableName=I_BT_PNT_Lo_ELEC
  P_cal1 : METI_Lib_vehicle_model/P_cal  Type_energy=電気  Type_output_energy=損失  Power_name=Pl_  t_Workspace_Name=BT_PNT_Lo_ELEC_LOSS  P_VariableName=Pl_BT_PNT_Lo_ELEC_LOSS  Across_VariableName=V_BT_PNT_Lo_ELEC_LOSS  Throgh_VariableName=I_BT_PNT_Lo_ELEC_LOSS
  SOC_MAX(%) : Constant  Value=BT_PNT_Lo_SOC_MAX_lo_batt
  SOC_MIN(%) : Constant  Value=BT_PNT_Lo_SOC_MIN_lo_batt
  SOC_START(%) : Constant  Value=BT_PNT_Lo_SOC_START_lo_batt
  Subsystem : Subsystem
  Sum : Sum  Inputs=|++
  Sum1 : Sum  Inputs=+-
  Sum2 : Sum
  Terminator1 : Terminator
  Terminator2 : Terminator
  map_OCV : Lookup  InputValues=BT_PNT_Lo_ocv_SOC_lo_batt_OCV_V_table_x_SOC  Table=BT_PNT_Lo_ocv_SOC_lo_batt_OCV_V_table  LookUpMeth=Interpolation-Use End Values
  sensor_BT_PNT_Lo : Outport
  volt_BT_PNT_Lo_V : Outport  Port=2
  tag scope: tScope_SOC_Batt=global
  wires:
  Sum/1 -> Memory6/1
  Capa_batt(Ah)/1 -> Cal_SOC/2(Capa_batt)
  SOC_START(%)/1 -> Cal_SOC/3(SOC_st)
  SOC_MAX(%)/1 -> Cal_SOC/4(SOC_MAX)
  SOC_MIN(%)/1 -> Cal_SOC/5(SOC_MIN)
  Memory6/1 -> volt_BT_PNT_Lo_V/1, P_cal/1  "volt_BT_PNT_Lo_V"
  map_OCV/1 -> Sum/1
  Subsystem/1(V_BT_PNT_Lo_V) -> P_cal1/1, Sum/2
  P_cal/1 -> Terminator2/1
  P_cal1/1 -> Terminator1/1
  Cal_SOC/1(SOC_out) -> Bus Creator4/1, map_OCV/1, [tScope_SOC_Batt]  "SOC_BT_PNT_Lo_PCT"
  Memory/1 -> sensor_BT_PNT_Lo/1  "sensor_BT_PNT_Lo"
  Sum1/1 -> P_cal/2, P_cal1/2, Subsystem/1(I_BT_PNT_Lo_A), Cal_SOC/1(I_Lo_BT_PNT_A)  "Current_Chg_Lo_BT_A"
  Sum2/1 -> Sum1/2  "current_ACC_A"
  current_ALT_PNT_A/1 -> Sum1/1
  current_ST_PNT_A/1 -> Sum2/1
  current_EL_PNT_A/1 -> Sum2/2
  Bus Creator4/1 -> Memory/1

== system METI_Thermal_ver01_Jmaab_2018b_Intg_Mref/Vehicle/CNT ==
  note: Control Model
  note: Gtoto From Tag Visibility for CAN
  VL_sensor : Inport
  Driver_Input : Inport  Port=2
  ALT_CNT : Subsystem
  BK_CNT : Subsystem
  Bus Creator1 : BusCreator  Inputs=4
  Bus Selector : BusSelector  OutputSignals=sensor_ENG_PNT,sensor_TM_PNT,sensor_BT_PNT_Lo,sensor_VL_PNT,sensor_BK_PNT
  CAN : Subsystem
  ENG_CNT : Subsystem
  Goto Tag Visibility : GotoTagVisibility  GotoTag=ENG_CNT_CAN_Tx
  Goto Tag Visibility1 : GotoTagVisibility  GotoTag=TM_CNT_CAN_Tx
  Goto Tag Visibility2 : GotoTagVisibility  GotoTag=ALT_CNT_CAN_Rx
  Goto Tag Visibility3 : GotoTagVisibility  GotoTag=ENG_CNT_CAN_Rx
  Goto Tag Visibility4 : GotoTagVisibility  GotoTag=TM_CNT_CAN_Rx
  Goto Tag Visibility5 : GotoTagVisibility  GotoTag=BK_CNT_CAN_Tx
  TM_CNT : Subsystem
  CNT_out : Outport
  wires:
  Bus Creator1/1 -> CNT_out/1  "CNT_out"
  Bus Selector/4 -> BK_CNT/2(sensor_VL_PNT_BUS)  "<sensor_VL_PNT>"
  VL_sensor/1 -> Bus Selector/1
  Bus Selector/3 -> ALT_CNT/1(sensor_BT_PNT_Lo_BUS)  "<sensor_BT_PNT_Lo>"
  Bus Selector/2 -> TM_CNT/1(sensor_TM_PNT)  "<sensor_TM_PNT>"
  Bus Selector/1 -> ENG_CNT/2(sensor_ENG_PNT)  "<sensor_ENG_PNT>"
  ALT_CNT/1(ALT_CNT_out) -> Bus Creator1/3
  ENG_CNT/1(ENG_CNT_out) -> Bus Creator1/1
  TM_CNT/1(TM_CNT_out) -> Bus Creator1/2
  Driver_Input/1 -> BK_CNT/1(Driver_Input), ENG_CNT/1(Driver_Input)
  BK_CNT/1(BK_CNT_out) -> Bus Creator1/4
  Bus Selector/5 -> BK_CNT/3(sensor_BK_PNT)  "<sensor_BK_PNT>"

== system METI_Thermal_ver01_Jmaab_2018b_Intg_Mref/Vehicle/EL_PNT ==
  note: 低圧側電気負荷
  volt_BT_PNT_Lo_V : Inport
  Add : Sum  Inputs=+-
  Ground : Ground
  P_cal1 : METI_Lib_vehicle_model/P_cal  Type_energy=電気  Type_output_energy=損失  Power_name=Pl_  t_Workspace_Name=EL_PNT_ELEC_LOSS  P_VariableName=Pl_EL_PNT_ELEC_LOSS  Across_VariableName=V_EL_PNT_ELEC_LOSS  Throgh_VariableName=I_EL_PNT_ELEC_LOSS
  Product3 : Product  Inputs=*/  RndMeth=Zero
  Resistance2 : Constant  Value=EL_PNT_R_bodyelec_lo_ohm
  Terminator1 : Terminator
  current_EL_PNT_A : Outport
  wires:
  Product3/1 -> P_cal1/2, current_EL_PNT_A/1  "current_EL_PNT_A"
  volt_BT_PNT_Lo_V/1 -> Add/1
  Ground/1 -> Add/2
  Add/1 -> P_cal1/1, Product3/1
  Resistance2/1 -> Product3/2
  P_cal1/1 -> Terminator1/1

== system METI_Thermal_ver01_Jmaab_2018b_Intg_Mref/Vehicle/ENG_PNT ==
  ENG_CNT_out : Inport
  w_ENG_PNT_radps : Inport  Port=2
  T_ENGTH_PNT : Inport  Port=3
  Bus Creator : BusCreator  Inputs=3
  Bus Creator1 : BusCreator  Inputs=2
  Bus Selector : BusSelector  OutputSignals=T_ENGTH_PNT__Head_K,T_ENGTH_PNT_Oil_K,T_ENGTH_PNT_Coolant_K
  Bus Selector7 : BusSelector  OutputSignals=open_throttle_per,flag_fuelcut,flag_IdleStop,timing_ignition,K_Fuel
  ENG_Plant : Subsystem
  K->degC : Subsystem
  Memory : Memory
  sensor_ENG_PNT : Outport
  trq_ENG_PNT_Nm : Outport  Port=2
  PHI_ENG_PNT : Outport  Port=3
  wires:
  Memory/1 -> sensor_ENG_PNT/1  "sensor_ENG_PNT"
  w_ENG_PNT_radps/1 -> ENG_Plant/6(w_ENG_PNT_radps)
  ENG_Plant/1(n_eng_rpm) -> Bus Creator/1
  ENG_CNT_out/1 -> Bus Selector7/1
  Bus Selector7/1 -> ENG_Plant/1(open_throttle_per)  "<open_throttle_per>"
  Bus Selector7/2 -> ENG_Plant/2(flag_fuelcut)  "<flag_fuelcut>"
  Bus Selector7/3 -> ENG_Plant/3(flag_IdleStop)  "<flag_IdleStop>"
  Bus Selector7/4 -> ENG_Plant/4(timing_ignition)  "<timing_ignition>"
  ENG_Plant/2(fuel_consumption) -> Bus Creator/2
  Bus Selector7/5 -> ENG_Plant/5(K_Fuel)  "<K_Fuel>"
  ENG_Plant/5(PHI_ENG_PNT_Head_W) -> Bus Creator1/2
  T_ENGTH_PNT/1 -> Bus Selector/1
  ENG_Plant/3(trq_ENG_PNT_Nm) -> trq_ENG_PNT_Nm/1
  ENG_Plant/4(PHI_ENG_PNT_Oil_W) -> Bus Creator1/1
  Bus Creator1/1 -> PHI_ENG_PNT/1  "PHI_ENG_PNT"
  Bus Selector/1 -> ENG_Plant/7(T_ENG_Cylinder_Head_K)  "<T_ENGTH_PNT__Head_K>"
  Bus Selector/2 -> ENG_Plant/8(T_ENG_ENGOil_K)  "<T_ENGTH_PNT_Oil_K>"
  Bus Selector/3 -> K->degC/1(K)  "<T_ENGTH_PNT_Coolant_K>"
  K->degC/1(degC) -> Bus Creator/3  "T_ENGTH_PNT_Coolant_degC"
  Bus Creator/1 -> Memory/1

== system METI_Thermal_ver01_Jmaab_2018b_Intg_Mref/Vehicle/PTTH ==
  note: image(imread('picture\ラジエーター_02s.jpg'))
  note: image(imread('picture\image\エンジン03.jpg'))
  note: image(imread('picture\image\トランスミッション02.jpg'))
  ENG_CNT_out : Inport
  TM_CNT_out : Inport  Port=2
  PHI_ENG_PNT : Inport  Port=3
  PHI_TM_PNT_BUS : Inport  Port=4
  v_VL_PNT_mps : Inport  Port=5
  ATM_PNT : Subsystem
  DTTH_PNT : Subsystem
  ENGTH_PNT : Subsystem
  RDTH_PNT : Subsystem
  T_TMTH_PNT : Outport
  T_ENGTH_PNT : Outport  Port=2
  wires:
  ENG_CNT_out/1 -> ENGTH_PNT/1(ENG_CNT_out), RDTH_PNT/3(ENG_CNT_out)
  PHI_ENG_PNT/1 -> ENGTH_PNT/2(PHI_ENG_PNT)
  v_VL_PNT_mps/1 -> RDTH_PNT/4(v_VL_PNT_mps), DTTH_PNT/4(v_VL_PNT_mps)
  ENGTH_PNT/1(T_ENGTH_PNT) -> T_ENGTH_PNT/1
  ENGTH_PNT/4(T_ENG_RD) -> RDTH_PNT/2(T_ENG_RD)
  ENGTH_PNT/2(PHI_ENG_ATM) -> ATM_PNT/1(PHI_ENG_ATM)
  ATM_PNT/1(T_ATM_RD) -> RDTH_PNT/5(T_ATM_RD)
  ATM_PNT/2(T_ATM_ENG) -> ENGTH_PNT/4(T_ATM_ENG)
  RDTH_PNT/1(PHI_RD_ATM) -> ATM_PNT/3(PHI_RD_ATM)
  RDTH_PNT/2(PHI_RD_ENG) -> ENGTH_PNT/3(PHI_RD_ENG)
  TM_CNT_out/1 -> DTTH_PNT/2(TM_CNT_out)
  ENGTH_PNT/3(T_ENG_TM) -> DTTH_PNT/1(T_ENG_TM)
  ATM_PNT/3(T_ATM_TM) -> DTTH_PNT/6(T_ATM_TM)
  PHI_TM_PNT_BUS/1 -> DTTH_PNT/3(PHI_TM_PNT)
  DTTH_PNT/1(T_TMTH_PNT) -> T_TMTH_PNT/1
  DTTH_PNT/2(PHI_TM_ATM) -> ATM_PNT/2(PHI_TM_ATM)
  DTTH_PNT/4(PHI_TM_ENG) -> ENGTH_PNT/5(PHI_TM_ENG)
  DTTH_PNT/3(PHI_TM_RD) -> RDTH_PNT/1(PHI_TM_RD)
  RDTH_PNT/3(T_RD_TM) -> DTTH_PNT/5(T_RD_TM)

== system METI_Thermal_ver01_Jmaab_2018b_Intg_Mref/Vehicle/ST_PNT ==
  ENG_CNT_out : Inport
  w_ENG_PNT_radps : Inport  Port=2
  volt_BT_PNT_Lo_V : Inport  Port=3
  Bus Selector1 : BusSelector  OutputSignals=flag_ON_Starter
  Constant1 : Constant  Value=OFF
  Constant6 : Constant  Value=OFF
  Gain : Gain  Gain=1/ST_PNT_Starter_Res_ohm
  Switch : Switch  Criteria=u2 > Threshold  Threshold=0.5
  Terminator : Terminator
  trq__ST_PNT_Nm : Outport
  current_ST_PNT_A : Outport  Port=2
  wires:
  volt_BT_PNT_Lo_V/1 -> Switch/1
  Switch/1 -> Gain/1
  Gain/1 -> current_ST_PNT_A/1  "current_ST_PNT_A"
  Constant6/1 -> Switch/3
  Constant1/1 -> trq__ST_PNT_Nm/1  "trq__ST_PNT_Nm"
  w_ENG_PNT_radps/1 -> Terminator/1
  ENG_CNT_out/1 -> Bus Selector1/1
  Bus Selector1/1 -> Switch/2  "<flag_ON_Starter>"

== system METI_Thermal_ver01_Jmaab_2018b_Intg_Mref/Vehicle/TM_PNT ==
  TM_CNT_out : Inport
  trq_ENG_PNT_Nm : Inport  Port=2
  trq_ALT_PNT_Nm : Inport  Port=3
  trq__ST_PNT_Nm : Inport  Port=4
  w_TR_PNT_radps : Inport  Port=5
  T_TMTH_PNT : Inport  Port=6
  Memory : Memory
  Memory1 : Memory
  TM_PNT : ModelReference  ModelNameDialog=METI_TM_PNT  SimulationMode=Normal  ModelReferenceVersion=1.420
  sensor_TM_PNT : Outport
  w_ENG_PNT_radps : Outport  Port=2
  trq_DS_PNT_Nm : Outport  Port=3
  PHI_TM_PNT : Outport  Port=4
  tag scope: TM_PNT_Info=global
  wires:
  TM_CNT_out/1 -> TM_PNT/1
  trq_ENG_PNT_Nm/1 -> TM_PNT/2
  trq_ALT_PNT_Nm/1 -> TM_PNT/3
  trq__ST_PNT_Nm/1 -> TM_PNT/4
  w_TR_PNT_radps/1 -> TM_PNT/5
  T_TMTH_PNT/1 -> TM_PNT/6
  TM_PNT/1 -> Memory1/1
  TM_PNT/3 -> Memory/1
  TM_PNT/4 -> PHI_TM_PNT/1
  TM_PNT/2 -> trq_DS_PNT_Nm/1
  TM_PNT/5 -> [TM_PNT_Info]
  Memory/1 -> w_ENG_PNT_radps/1  "w_ENG_PNT_radps"
  Memory1/1 -> sensor_TM_PNT/1  "sensor_TM_PNT"

== system METI_Thermal_ver01_Jmaab_2018b_Intg_Mref/Vehicle/TR_PNT ==
  note: 転がり抵抗
  note: 並進⇔回転変換
  note: トルク⇔力変換
  note: omg (回転数rad/s) = v (車速m/s) / r (タイヤ半径(m))
  note: M (トルクNm) = F (力(N)） × r (タイヤ半径(m))
  note: 車両を動かす側が正
  note: 車両を動かす側が正
  trq_DF_PNT_Nm : Inport
  trq_BK_PNT_Nm : Inport  Port=2
  v_VL_PNT_mps : Inport  Port=3
  Constant2 : Constant  Value=1/tire_r
  Product5 : Product  RndMeth=Zero
  Product6 : Product  RndMeth=Zero
  Q_cal1 : METI_Lib_vehicle_model/P_cal  Commented=on  Type_energy=並進運動  Type_output_energy=出力  Power_name=Po_  t_Workspace_Name=TR_PNT_MECK_DN  P_VariableName=Po_TR_PNT_MECK_DN  Across_VariableName=v_TR_PNT_MECK_DN  Throgh_VariableName=F_TR_PNT_MECK_DN
  Q_cal2 : METI_Lib_vehicle_model/P_cal  Commented=on  Type_energy=回転運動  Type_output_energy=出力  Power_name=Po_  t_Workspace_Name=TR_PNT_MECK_UP  P_VariableName=Po_TR_PNT_MECK_UP  Across_VariableName=w_TR_PNT_MECK_UP  Throgh_VariableName=tq_TR_PNT_MECK_UP
  Subtract2 : Sum
  Sum2 : Sum  Inputs=-+
  Terminator1 : Terminator  Commented=on
  Terminator2 : Terminator  Commented=on
  cal_roll_resi : METI_Lib_vehicle_model/vehicle_model/cal_roll_resi  Myu_tire=myu  Vehicle_Mass=M  Gravi_acc=g
  f_TR_PNT_N : Outport
  w_TR_PNT_radps : Outport  Port=2
  wires:
  Sum2/1 -> f_TR_PNT_N/1  "f_TR_PNT_N"
  cal_roll_resi/1 -> Sum2/1, Q_cal1/2
  Product6/1 -> Sum2/2, Q_cal2/2
  Q_cal1/1 -> Terminator1/1
  Constant2/1 -> Product6/1, Product5/2
  v_VL_PNT_mps/1 -> Product5/1, cal_roll_resi/1, Q_cal1/1, Q_cal2/1
  Q_cal2/1 -> Terminator2/1
  Product5/1 -> w_TR_PNT_radps/1  "w_TR_PNT_radps"
  Subtract2/1 -> Product6/2  "trq_TR_in_Nm"
  trq_BK_PNT_Nm/1 -> Subtract2/2
  trq_DF_PNT_Nm/1 -> Subtract2/1

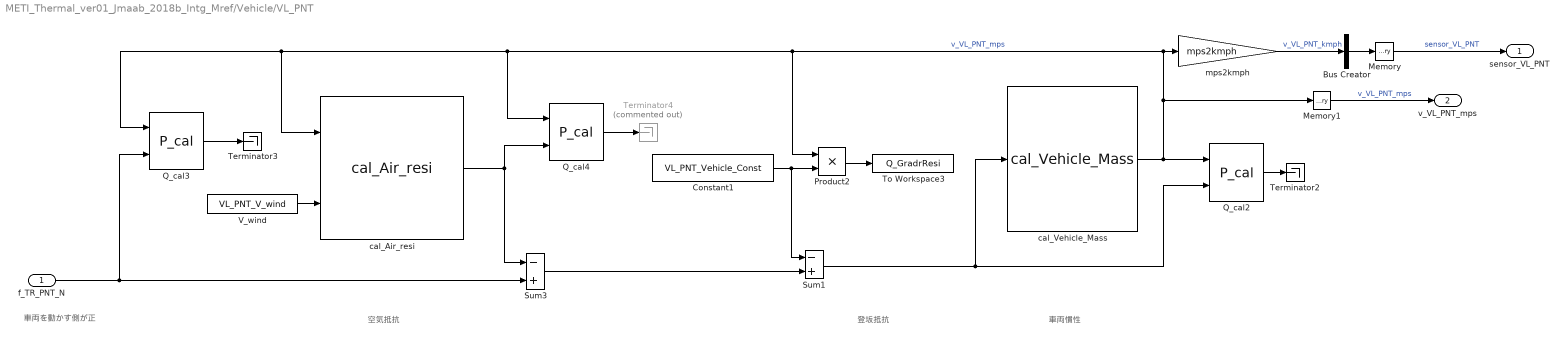
== system METI_Thermal_ver01_Jmaab_2018b_Intg_Mref/Vehicle/VL_PNT ==
  note: 空気抵抗
  note: 車両慣性
  note: 登坂抵抗
  note: 車両を動かす側が正
  f_TR_PNT_N : Inport
  Bus Creator : BusCreator  Inputs=1
  Constant1 : Constant  Value=VL_PNT_Vehicle_Const
  Memory : Memory
  Memory1 : Memory
  Product2 : Product
  Q_cal2 : METI_Lib_vehicle_model/P_cal  Type_energy=並進運動  Type_output_energy=出力  Power_name=Po_  t_Workspace_Name=VL_PNT_MASS_MECK  P_VariableName=Po_VL_PNT_MASS_MECK  Across_VariableName=v_VL_PNT_MASS_MECK  Throgh_VariableName=F_VL_PNT_MASS_MECK
  Q_cal3 : METI_Lib_vehicle_model/P_cal  Type_energy=並進運動  Type_output_energy=出力  Power_name=Po_  t_Workspace_Name=VL_PNT_MECK  P_VariableName=Po_VL_PNT_MECK  Across_VariableName=v_VL_PNT_MECK  Throgh_VariableName=F_VL_PNT_MECK
  Q_cal4 : METI_Lib_vehicle_model/P_cal  Type_energy=並進運動  Type_output_energy=損失  Power_name=Pl_  t_Workspace_Name=VL_PNT_Airresi_MECK_LOSS  P_VariableName=Pl_VL_PNT_Airresi_MECK_LOSS  Across_VariableName=v_VL_PNT_Airresi_MECK_LOSS  Throgh_VariableName=F_VL_PNT_Airresi_MECK_LOSS
  Sum1 : Sum  Inputs=-+
  Sum3 : Sum  Inputs=-+
  Terminator2 : Terminator
  Terminator3 : Terminator
  Terminator4 : Terminator  Commented=on
  To Workspace3 : ToWorkspace  VariableName=Q_GradrResi  SaveFormat=Structure With Time  SampleTime=-1
      settings: Decimation=100
  V_wind : Constant  Value=VL_PNT_V_wind
  cal_Air_resi : METI_Lib_vehicle_model/vehicle_model/cal_Air_resi  Vel_max=vel_max
  cal_Vehicle_Mass : METI_Lib_vehicle_model/vehicle_model/cal_Vehicle_Mass  Vehicle_Mass=M
  mps2kmph : Gain  Gain=mps2kmph
  sensor_VL_PNT : Outport
  v_VL_PNT_mps : Outport  Port=2
  wires:
  Product2/1 -> To Workspace3/1
  Sum3/1 -> Sum1/2
  Sum1/1 -> Q_cal2/2, cal_Vehicle_Mass/1
  cal_Vehicle_Mass/1 -> Memory1/1, Q_cal3/1, cal_Air_resi/1, Q_cal4/1, Product2/1, mps2kmph/1, Q_cal2/1  "v_VL_PNT_mps"
  cal_Air_resi/1 -> Q_cal4/2, Sum3/1
  V_wind/1 -> cal_Air_resi/2
  Constant1/1 -> Sum1/1, Product2/2
  Q_cal2/1 -> Terminator2/1
  Q_cal3/1 -> Terminator3/1
  Q_cal4/1 -> Terminator4/1
  mps2kmph/1 -> Bus Creator/1  "v_VL_PNT_kmph"
  f_TR_PNT_N/1 -> Sum3/2, Q_cal3/2
  Bus Creator/1 -> Memory/1
  Memory/1 -> sensor_VL_PNT/1  "sensor_VL_PNT"
  Memory1/1 -> v_VL_PNT_mps/1  "v_VL_PNT_mps"

== system METI_Thermal_ver01_Jmaab_2018b_Intg_Mref/Driver/Caliculate_Opeining_Accel/FB ==
  delta_v_VL_kmph : Inport
  Acc_D_Gain : Gain  Gain=D_Gain
  Acc_I_Gain : Gain  Gain=I_Gain
  Acc_P_Gain : Gain  Gain=P_Gain
  Acc_P_Gain1 : Gain  Gain=P_Gain
  Derivative : Derivative
  Filter : Subsystem  Commented=through
  Integrator : Integrator
  Memory : Memory
  Product1 : Product
  Saturation2 : Saturate  UpperLimit=1  LowerLimit=0
  Sum : Sum  Inputs=+++
  Terminator : Terminator
  FB_open_accel_per : Outport
  wires:
  Filter/1(Out1) -> Product1/2
  Saturation2/1 -> Acc_P_Gain/1
  Acc_P_Gain/1 -> Product1/1
  Sum/1 -> FB_open_accel_per/1
  Derivative/1 -> Acc_D_Gain/1
  Integrator/1 -> Acc_I_Gain/1
  delta_v_VL_kmph/1 -> Memory/1
  Acc_I_Gain/1 -> Sum/3
  Acc_D_Gain/1 -> Sum/2
  Product1/1 -> Sum/1
  Memory/1 -> Saturation2/1, Filter/1(In1), Acc_P_Gain1/1, Integrator/1, Derivative/1
  Acc_P_Gain1/1 -> Terminator/1

== system METI_Thermal_ver01_Jmaab_2018b_Intg_Mref/Driver/Caliculate_Opeining_Accel/FF ==
  note: 速度とパワーでF/B出来るようにモデルを用意しておく
      | 切り替えスイッチを作っておく
  v_VL_PNT_kmph : Inport
  target_v_VL_kmph : Inport  Port=2
  pre_n_eng_rpm : Inport  Port=3
  pre_ratio_CVT : Inport  Port=4
  Air_Resistance : Subsystem
  Cal_M_ENG_jiku2 : Subsystem
  Constant1 : Constant  Value=TM_CNT_CVT_ratio_LL
  Constant3 : Constant  Value=tire_r
  Constant4 : Constant  Value=DF_PNT_DF_gear
  Inertial_Resistance : Subsystem
  MinMax : MinMax  Function=max  Inputs=2
  Product8 : Product  Inputs=*/*/  RndMeth=Zero
  Rolling_Resistance : Subsystem
  Sum4 : Sum  Inputs=+++
  Terminator : Terminator
  Transfer Fcn : TransferFcn  Denominator=[TM_PNT_Tau_CVT_ratio_s 1]
  kmph2mps : Gain  Gain=kmph2mps
  kmph2mps1 : Gain  Gain=kmph2mps
  FF_open_accel_per : Outport
  wires:
  kmph2mps/1 -> Inertial_Resistance/1(V_tgt), Rolling_Resistance/1(V_tgt), Air_Resistance/1(V_tgt)
  target_v_VL_kmph/1 -> kmph2mps/1
  Sum4/1 -> Product8/1
  Constant4/1 -> Product8/2
  Constant3/1 -> Product8/3
  Air_Resistance/1(F_air_resi) -> Sum4/2
  Rolling_Resistance/1(F_rollresi) -> Sum4/3
  Inertial_Resistance/1(F_Inertia) -> Sum4/1
  pre_ratio_CVT/1 -> Transfer Fcn/1
  Constant1/1 -> MinMax/2
  MinMax/1 -> Product8/4
  Transfer Fcn/1 -> MinMax/1
  v_VL_PNT_kmph/1 -> kmph2mps1/1
  kmph2mps1/1 -> Terminator/1
  Cal_M_ENG_jiku2/1(FF_open_accel_per) -> FF_open_accel_per/1
  Product8/1 -> Cal_M_ENG_jiku2/1(FF_trq_accel_Nm)  "FF_trq_accel_Nm"
  pre_n_eng_rpm/1 -> Cal_M_ENG_jiku2/2(pre_n_eng_rpm)

== system METI_Thermal_ver01_Jmaab_2018b_Intg_Mref/Vehicle/ALT_PNT/Subsystem ==
  note: V_ALT_PNT
  note: オルタ要求トルク上限/下限ガード処理追加
      | (低回転数、低電流時に要求トルクが過大となるのを防止するため
      |  :マップの外挿方法が線形となっていることが原因)
  target_volt_ALT_V : Inport
  w_ROT_slavepulley12 : Inport  Port=2
  volt_BT_PNT_Lo_V : Inport  Port=3
  Constant1 : Constant  Value=ALT_PNT_ALT_GDCurrent_A
  Constant2 : Constant  Value=ALT_PNT_ALT_GDVolt_V
  I_alt_cal : Subsystem
  Torque_Guard : Subsystem
  Transfer Fcn1 : TransferFcn  Denominator=|
      | [ALT_PNT_Tau_Alternator_trq_Nm
      |  1]
  omg2rpm : Gain  Gain=radpsec2rpm
  current_ALT_PNT_A : Outport
  trq_trqsource : Outport  Port=2
  wires:
  I_alt_cal/1(I_alt) -> Torque_Guard/1(current_ALT_PNT_A), current_ALT_PNT_A/1  "current_ALT_PNT_A"
  target_volt_ALT_V/1 -> I_alt_cal/1(target_volt_ALT_V)
  volt_BT_PNT_Lo_V/1 -> Torque_Guard/2(V_ALT_PNT), I_alt_cal/2(volt_BT_PNT_Lo_V)
  Transfer Fcn1/1 -> trq_trqsource/1
  omg2rpm/1 -> Torque_Guard/3(n_ROT_slavepulley12_rpm), I_alt_cal/3(rpm_alt)  "n_ROT_slavepulley12_rpm"
  w_ROT_slavepulley12/1 -> omg2rpm/1
  Constant1/1 -> Torque_Guard/4(ALT_GDCurrent)
  Constant2/1 -> Torque_Guard/5(ALT_GDVolt)
  Torque_Guard/1(trq_trqsource) -> Transfer Fcn1/1

== system METI_Thermal_ver01_Jmaab_2018b_Intg_Mref/Vehicle/ALT_PNT/pulley_slave ==
  note: プーリー比
  note: プーリー効率
  w_ENG_PNT_radps : Inport
  trq_slavepulley12 : Inport  Port=2
  P_cal : AZAPA_Lib_vehicle_model/P_cal  Commented=on  Type_energy=並進運動  Type_output_energy=出力  Power_name=Po_  t_Workspace_Name=MOTOR_MECK  P_VariableName=Po_MOTOR_MECK  Across_VariableName=v_MOTOR_MECK  Throgh_VariableName=F_MOTOR_MECK
  Product : Product  RndMeth=Zero
  Product1 : Product  RndMeth=Zero
  eta_cal2 : METI_Lib_vehicle_model/eta_cal2  SystemSampleTime=-1
  eta_pulley : Constant  Value=ALT_PNT_eta_pulley_alt
  ratio_pulley : Constant  Value=ALT_PNT_ratio_pulley_alt
  trq_slavepulley11 : Outport
  w_slavepulley12 : Outport  Port=2
  tag scope: tScope_pulley1Loss=global
  wires:
  eta_cal2/1 -> P_cal/2
  P_cal/1 -> [tScope_pulley1Loss]
  w_ENG_PNT_radps/1 -> P_cal/1, Product1/1
  eta_cal2/2 -> trq_slavepulley11/1
  trq_slavepulley12/1 -> Product/2
  eta_pulley/1 -> eta_cal2/1
  Product1/1 -> w_slavepulley12/1
  ratio_pulley/1 -> Product/1, Product1/2
  Product/1 -> eta_cal2/2

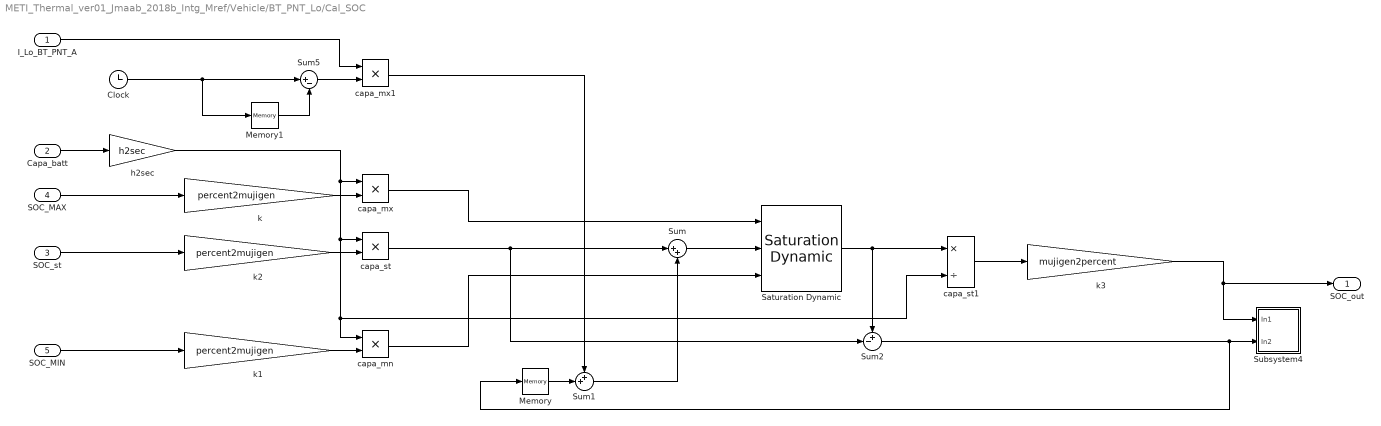
== system METI_Thermal_ver01_Jmaab_2018b_Intg_Mref/Vehicle/BT_PNT_Lo/Cal_SOC ==
  I_Lo_BT_PNT_A : Inport
  Capa_batt : Inport  Port=2
  SOC_st : Inport  Port=3
  SOC_MAX : Inport  Port=4
  SOC_MIN : Inport  Port=5
  Clock : Clock
  Memory : Memory
  Memory1 : Memory
  Saturation Dynamic : simulink/Discontinuities/Saturation Dynamic  OutMin=[]  OutMax=[]  OutDataTypeStr=Inherit: Same as second input  OutDataType=fixdt(1, 16)  OutScaling=2^-10  DoSatur=off
  Subsystem4 : Subsystem  mask{SOC=SOC_LoBat, VariableName=Asec_LoBat}
      mask prompts: SOC "バッテリSOC"; VariableName "バッテリ容量変化量(Asec)"
  Sum : Sum  Inputs=|++
  Sum1 : Sum  Inputs=++|
  Sum2 : Sum  Inputs=+-|
  Sum5 : Sum  Inputs=|+-
  capa_mn : Product  RndMeth=Zero
  capa_mx : Product  RndMeth=Zero
  capa_mx1 : Product  RndMeth=Zero
  capa_st : Product  RndMeth=Zero
  capa_st1 : Product  Inputs=*/  RndMeth=Zero
  h2sec : Gain  Gain=h2sec
  k : Gain  Gain=percent2mujigen
  k1 : Gain  Gain=percent2mujigen
  k2 : Gain  Gain=percent2mujigen
  k3 : Gain  Gain=mujigen2percent
  SOC_out : Outport
  wires:
  Sum5/1 -> capa_mx1/2
  Memory1/1 -> Sum5/2
  Sum/1 -> Saturation Dynamic/2
  Clock/1 -> Sum5/1, Memory1/1
  capa_mx1/1 -> Sum1/1
  k3/1 -> Subsystem4/1(In1), SOC_out/1
  Sum1/1 -> Sum/2
  Memory/1 -> Sum1/2
  k2/1 -> capa_st/2
  k1/1 -> capa_mn/2
  k/1 -> capa_mx/2
  capa_st/1 -> Sum2/2, Sum/1
  Saturation Dynamic/1 -> Sum2/1, capa_st1/1
  capa_mx/1 -> Saturation Dynamic/1
  capa_mn/1 -> Saturation Dynamic/3
  capa_st1/1 -> k3/1
  h2sec/1 -> capa_mn/1, capa_st1/2, capa_st/1, capa_mx/1
  SOC_MIN/1 -> k1/1
  SOC_MAX/1 -> k/1
  SOC_st/1 -> k2/1
  Capa_batt/1 -> h2sec/1
  I_Lo_BT_PNT_A/1 -> capa_mx1/1
  Sum2/1 -> Memory/1, Subsystem4/2(In2)

== system METI_Thermal_ver01_Jmaab_2018b_Intg_Mref/Vehicle/BT_PNT_Lo/Subsystem ==
  I_BT_PNT_Lo_A : Inport
  Divide : Product
  Resistivity : Constant  Value=BT_PNT_Lo_R_lo_batt_ohm
  Sum : Sum  Inputs=|++
  Transfer Fcn : TransferFcn  Numerator=[0.01]  Denominator=[0.1 1]
  V_BT_PNT_Lo_V : Outport
  wires:
  Resistivity/1 -> Divide/2
  Divide/1 -> Sum/1
  I_BT_PNT_Lo_A/1 -> Divide/1, Transfer Fcn/1
  Sum/1 -> V_BT_PNT_Lo_V/1
  Transfer Fcn/1 -> Sum/2

== system METI_Thermal_ver01_Jmaab_2018b_Intg_Mref/Vehicle/CNT/ALT_CNT ==
  sensor_BT_PNT_Lo_BUS : Inport
  ALT_Ctrl : Subsystem
  Bus Creator6 : BusCreator  Inputs=1
  Bus Selector1 : BusSelector  OutputSignals=flag_fuelcut,flag_IdleStop,n_eng_rpm
  Bus Selector9 : BusSelector  OutputSignals=SOC_BT_PNT_Lo_PCT
  ALT_CNT_out : Outport
  wires:
  [ALT_CNT_CAN_Rx] -> Bus Selector1/1
  Bus Selector1/1 -> ALT_Ctrl/2(flag_fuelcut)  "<flag_fuelcut>"
  Bus Selector1/2 -> ALT_Ctrl/3(flag_IdleStop)  "<flag_IdleStop>"
  Bus Selector1/3 -> ALT_Ctrl/4(n_eng_rpm)  "<n_eng_rpm>"
  ALT_Ctrl/1(target_volt_ALT_V) -> Bus Creator6/1
  sensor_BT_PNT_Lo_BUS/1 -> Bus Selector9/1
  Bus Selector9/1 -> ALT_Ctrl/1(SOC_BT_PNT_Lo_PCT)  "<SOC_BT_PNT_Lo_PCT>"
  Bus Creator6/1 -> ALT_CNT_out/1  "ALT_CNT_out"

== system METI_Thermal_ver01_Jmaab_2018b_Intg_Mref/Vehicle/CNT/BK_CNT ==
  Driver_Input : Inport
  sensor_VL_PNT_BUS : Inport  Port=2
  sensor_BK_PNT : Inport  Port=3
  BK_Ctrl : Subsystem
  Bus Creator1 : BusCreator  Inputs=1
  Bus Creator2 : BusCreator  Inputs=2
  Bus Selector1 : BusSelector  OutputSignals=trq_BK_PNT_Nm
  Bus Selector12 : BusSelector  OutputSignals=v_VL_PNT_kmph
  Bus Selector4 : BusSelector  OutputSignals=open_brake_per
  BK_CNT_out : Outport
  tag scope: BK_CNT_CAN_Tx=scoped
  wires:
  BK_Ctrl/2(v_VL_PNT_kmph) -> Bus Creator2/1
  Bus Selector12/1 -> BK_Ctrl/2(v_VL_PNT_kmph_in)  "<v_VL_PNT_kmph>"
  sensor_VL_PNT_BUS/1 -> Bus Selector12/1
  BK_Ctrl/3(trq_BK_PNT_Nm) -> Bus Creator2/2
  Bus Creator2/1 -> [BK_CNT_CAN_Tx]  "BK_CNT_CAN_Tx"
  Bus Selector1/1 -> BK_Ctrl/3(trq_BK_PNT_Nm_in)  "<trq_BK_PNT_Nm>"
  sensor_BK_PNT/1 -> Bus Selector1/1
  Bus Creator1/1 -> BK_CNT_out/1  "BK_CNT_out"
  Bus Selector4/1 -> BK_Ctrl/1(open_brake_per_in)  "<open_brake_per>"
  Driver_Input/1 -> Bus Selector4/1
  BK_Ctrl/1(open_brake_per) -> Bus Creator1/1

== system METI_Thermal_ver01_Jmaab_2018b_Intg_Mref/Vehicle/CNT/CAN ==
  note: CAN Bus Model
  ALT_CNT : Subsystem
  BK_CNT : Subsystem
  ENG_CNT : Subsystem
  Pwtr_CAN : Subsystem
  TM_CNT : Subsystem
  wires:
  Pwtr_CAN/1(Pwtr_CAN) -> BK_CNT/1(Pwtr_CAN), ALT_CNT/1(Pwtr_CAN), ENG_CNT/1(Pwtr_CAN), TM_CNT/1(Pwtr_CAN)
  ENG_CNT/1(ENG_CNT_CAN_Tx) -> Pwtr_CAN/1(ENG_CNT_CAN_Tx)
  TM_CNT/1(TM_CNT_CAN_Tx) -> Pwtr_CAN/2(TM_CNT_CAN_Tx)
  BK_CNT/1(BK_CNT_CAN_Tx) -> Pwtr_CAN/3(BK_CNT_CAN_Tx)
